simulink model "Junctions3"  (Simulink 8.7)
settings: Solver=ode45  StartTime=0.0  StopTime=10.0  RelTol=1e-3
settings Model: Creator=scaife  LastModifiedBy=bourbouh  ExtModeAutoUpdateStatusClock=off
settings DataIOCC: SignalLoggingSaveFormat=ModelDataLogs  SignalLoggingName=sigsOut
settings DebuggingCC: SaveWithParameterizedLinksMsg=none  SignalResolutionControl=TryResolveAllWithWarning  MultiTaskDSMMsg=warning  MultiTaskCondExecSysMsg=none  StrictBusMsg=None
settings HardwareCC: TargetUnknown=on
settings SFSimCC: SimParseCustomCode=off
settings GRTTargetCC: GeneratePreprocessorConditionals=Use local settings  CombineOutputUpdateFcns=off  GRTInterface=on

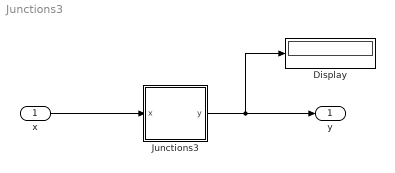
== system Junctions3 ==
  x : Inport
  Display : Display
  Junctions3 : Stateflow chart  TreatAsAtomicUnit=on
  y : Outport
  wires:
  x/1 -> Junctions3/1(x)
  Junctions3/1(y) -> y/1, Display/1

== stateflow chart Junctions3 ==
  state A
  state B
  (default) -> A
  A -> (junction 7) : [x==0]{y=0}
  (junction 7) -> (junction 8) : [y==0]{y++}
  (junction 8) -> (junction 9) : [y==1]{y++}
  (junction 9) -> (junction 10) : [y==2]{y++}
  (junction 10) -> B : {y++}
  data: x input int32; y output int32 =111111
